simulink model "sim_7"  (R2015b)
settings: Solver=ode45  StartTime=0  StopTime=1000  FixedStep=1e-3  RelTol=1e-4
undefined symbols (not defined in the file or in its folder): alpha_nc, alpha_nw, B, currentCoeffMatrix, D, E, f, h, H, K2_np, K3_np, K4_np, Kd_surge, Kd_sway, Kd_yaw, Ki_surge, Ki_sway, Ki_yaw, Kp_surge, Kp_sway, Kp_yaw, M_inverse, mu, N_freq, P0, Par, phi, Q, R, S, Sim, T_pinv, TA_sampling_time, thrusterPositionX, thrusterPositionY, thrusters, thrustersInitialAlpha, U_mean_c, U_mean_w, windCoeffMatrix, x0
libraries: simulink_extras x8, marine_gnc x5, simulink x5
(part 2 of 2)

== matlab function sim_7/Env_NEW/get wind coeffcients ==
  data: alpha input; C output; windCoeffMatrix input
function C   = WindCoeffcients(alpha, windCoeffMatrix)
% Initialization of the return parameter
C=zeros(6,1);

while alpha > 360
    alpha = alpha - 360;
end

while alpha < 0
    alpha = alpha + 360;
end

alpha_mod = mod(alpha,10);
avrundet_alpha = alpha - alpha_mod;
index = avrundet_alpha/10+1;

C1 = windCoeffMatrix(index,:)';
C2 = windCoeffMatrix(index+1,:)';

for i = 1:6
    diff = C2(i)-C1(i);
    point = (diff/10)*alpha_mod;
    C(i) = C1(i)+point;
end

end
